simulink model "PushButton"  (R2018a)
settings: Solver=FixedStepAuto  StartTime=0.0  StopTime=inf  FixedStep=.001  RelTol=1e-3  EnableMultiTasking=on
libraries: arduinolib x2, simulink x1
settings Model: ExtModeTrigDuration=2  Creator=jonathancoulter  LastModifiedBy=jonathancoulter
settings SolverCC: AutoInsertRateTranBlk=on
settings OptimizationCC: DefaultParameterBehavior=Inlined  UseFloatMulNetSlope=on  InlineInvariantSignals=on  PassReuseOutputArgsThreshold=0  EfficientFloat2IntCast=on  MaxStackSize=64
settings DebuggingCC: ParameterTunabilityLossMsg=error
settings HardwareCC: ProdBitPerInt=16  ProdBitPerPointer=16  ProdBitPerSizeT=16  ProdBitPerPtrDiffT=16  ProdLargestAtomicFloat=None  ProdWordSize=8  ProdHWDeviceType=Atmel->AVR  UseEmbeddedCoderFeatures=off
settings SFSimCC: MATLABDynamicMemAlloc=off
settings RTWCC: SystemTargetFile=ert.tlc  HardwareBoard=Arduino Mega 2560  TLCOptions=-aInlineSetEventsForThisBaseRateFcn=TLC_FALSE -aSuppressMultiTaskScheduler=TLC_FALSE -aRateBasedStepFcn=1  TemplateMakefile=ert_default_tmf  Toolchain=Arduino AVR  BuildConfiguration=Faster Runs  CheckMdlBeforeBuild=Warning
settings CodeAppCC: ForceParamTrailComments=on  OperatorAnnotations=on  StateflowObjectComments=on  MATLABSourceComments=on
settings ERTTargetCC: ERTCustomFileBanners=off  SupportNonFinite=off  SupportContinuousTime=on  SupportNonInlinedSFcns=on  RemoveResetFunc=off  SupportVariableSizeSignals=on  ModelStepFunctionPrototypeControlCompliant=off  InlinedParameterPlacement=NonHierarchical

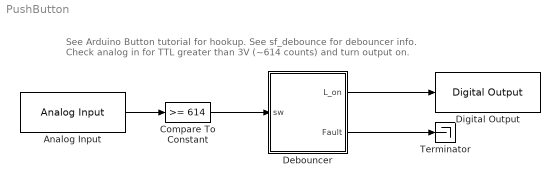
== system PushButton ==
  note: See Arduino Button tutorial for hookup. See sf_debounce for debouncer info.
      | Check analog in for TTL greater than 3V (~614 counts) and turn output on.
  Analog Input : arduinolib/Analog Input  pinNumber=0  ReadResultsOnly=off  ConversionTriggerSource=Software  ExternalTriggerType=uint32(0)  OutputDataType=uint16  EnableConversionCompleteNotify=off  EnableOuputStatus=off  SampleTime=-1  blockPlatform=arduino
  Compare To Constant : simulink/Logic and Bit Operations/Compare To Constant  relop=>=  const=614  OutDataTypeStr=boolean
  Debouncer : Stateflow chart  TreatAsAtomicUnit=on
  Digital Output : arduinolib/Digital Output  pinNumber=13  blockPlatform=arduino
  Terminator : Terminator
  wires:
  Analog Input/1 -> Compare To Constant/1
  Debouncer/1(L_on) -> Digital Output/1
  Debouncer/2(" Fault") -> Terminator/1
  Compare To Constant/1 -> Debouncer/1(sw)

== stateflow chart PushButton/Debouncer ==
  settings: updateMethod=DISCRETE  sampleTime=0.001
  state Off
    en: L_on = false;
    state Fault
      % Isolation
    state Normal
    Fault -> Normal : % Recovery
        | after(1, sec)
    (default) -> Normal
  state Debounce
    state Off
    state On
    Debounce.Off -> Debounce.On [order 2] : [sw == true]
    Debounce.On -> Debounce.Off [order 2] : [sw == false]
  state On
    en: L_on = true;
  (default) -> Off
  Normal -> Debounce.On : [sw == true]
  Debounce -> Fault : % Detection
      | after(0.3, sec)
  Debounce.Off -> Off [order 1] : after(0.1, sec)
  Debounce.On -> On [order 1] : after(0.1, sec)
  On -> Debounce.Off : [sw == false]
  data: sw input; L_on output boolean =false; Fault output boolean
